simulink model "simulation"  (R2021b)
settings: Solver=ode15s  StartTime=0  StopTime=2474  RelTol=1e-4
model workspace: external: MATLAB File Z:\sleipner_simulation\data.m (data not in the file)
values from neighbouring files (symbols this model uses):
  AccessoryLoad = 200    [data.m]
  aeroDragCoeff = 0.38    [data.m]
  airDensity = 1.23    [data.m]
  C = 628.297    [data.m]
  driveLineGear = 3.55    [data.m]
  energyCapacity = 40    [data.m]
  frontArea = 16    [data.m]
  gravity = 9.82    [data.m]
  inertialMassVeh = 5000    [data.m]
  initialSOC = 0.95    [data.m]
  InternalResistance = 0.1    [data.m]
  kc = 0.0452    [data.m]
  ki = 0.0167    [data.m]
  kw = 5.664E-6    (= 5.664e-06)    [data.m]
  massVeh = 5000    [data.m]
  maxBreakForce = 10000    [data.m]
  motorModelMaxPowerOut = 10000    [data.m]
  motorModelMaxTrqOut = 600    [data.m]
  openCircuitVoltage = 396    [data.m]
  regenbreakFraction = 0.55    [data.m]
  rollingResistCoeff = 0.01    [data.m]
  spinLoss = 6    [data.m]
  wheelRadius = 0.35    [data.m]
undefined symbols (not defined in the file or in its folder): magnitude
libraries: simulink x5, slpidlib x1, autolibshared x1
settings Model: Creator=alexa  LastModifiedBy=alebostr
settings DebuggingCC: UnconnectedInputMsg=none  UnconnectedOutputMsg=none  UnconnectedLineMsg=none  UnderSpecifiedDimensionMsg=warning
settings ModelReferenceCC: EnableRefExpFcnMdlSchedulingChecks=off
settings RTWCC: DLArmComputeVersion=20.02.1

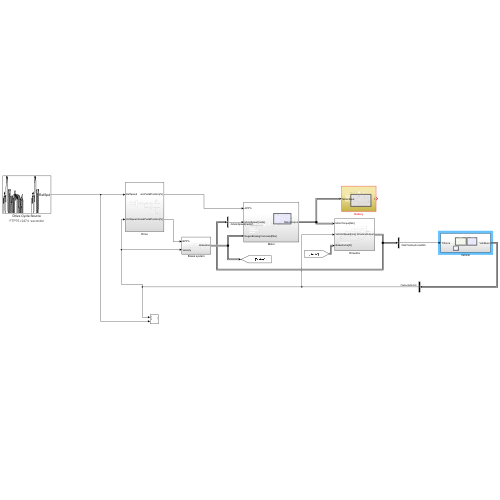
[thumbnail: Simulink's stored preview of the top-level diagram]
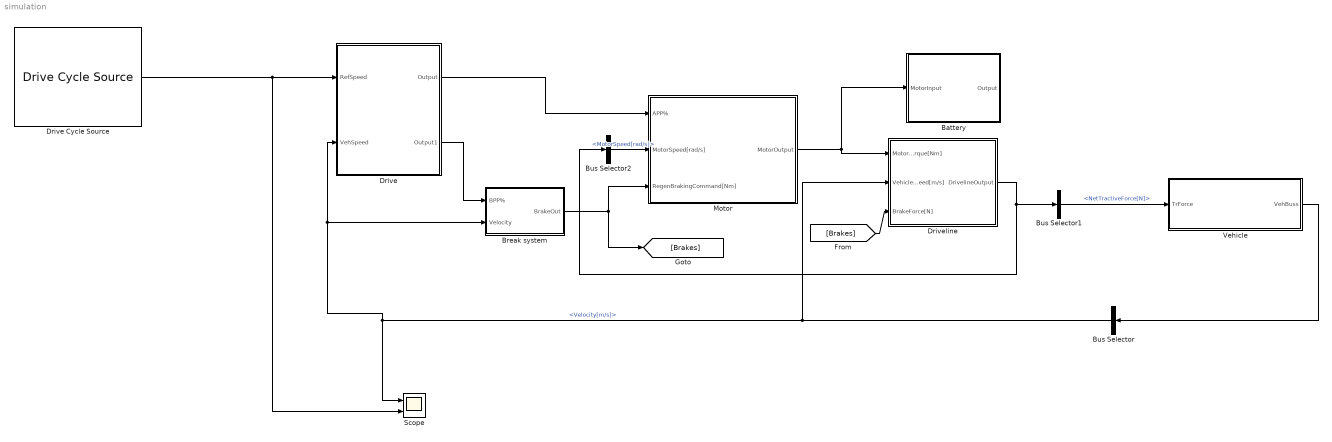
== system simulation ==
  Battery : Subsystem
  Break system : Subsystem
  Bus Selector : BusSelector  OutputSignals=Velocity[m/s]
  Bus Selector1 : BusSelector  OutputSignals=NetTractiveForce[N]
  Bus Selector2 : BusSelector  OutputSignals=MotorSpeed[rad/s]
  Drive : Subsystem
  Drive Cycle Source : autolibshared/Drive Cycle Source  cycleVar=FTP75  fileVar=cycleFTP75.mat  tfinal="2474  seconds"  cycleRepeat=off  outAccPort=off  outGearPort=off  gearList=No gear data  t_wot1=5  xdot_woto=0  xdot_wot1=30  t_wot2=20  xdot_wot2=0  t_wotend=30  srcUnit=m/s  outUnit=m/s  srcAccUnit=m/s/s  outAccUnit=m/s^2  dt=0  aMode=1  faultOption=off  velBnd=2  velBndUnit=mph  inUnit=m/s  timeBnd=1  failOption=off  stopSim=off  maxFaultCnt=10  maxFaultTime=2  maxTotFaultTime=15  traceOption=off  dtTrace=1  traceWindow=10  lastDCname=FTP75  lastOutUnit=mph  lastDT=0  lastTB=1  lastSB=2  forceCalcBound=off
      settings: SourceProductBaseCode=PW,DR,MT,UV,VE
  Driveline : Subsystem
  Motor : Subsystem
  Scope : Scope  NumInputPorts=2
  Vehicle : Subsystem
  wires:
  Drive/2(Output1) -> Break system/1(BPP%)
  Break system/1(BrakeOut) -> [Brakes], Motor/3(RegenBrakingCommand[Nm])
  Drive/1(Output) -> Motor/1(APP%)
  [Brakes] -> Driveline/3(BrakeForce[N])
  Motor/1(MotorOutput) -> Driveline/1(MotorTorque[Nm]), Battery/1(MotorInput)
  Driveline/1(DrivelineOutput) -> Bus Selector1/1, Bus Selector2/1
  Bus Selector2/1 -> Motor/2(MotorSpeed[rad/s])  "<MotorSpeed[rad/s]>"
  Vehicle/1(VehBuss) -> Bus Selector/1
  Bus Selector/1 -> Driveline/2(VehicleSpeed[m/s]), Drive/2(VehSpeed), Break system/2(Velocity), Scope/1  "<Velocity[m/s]>"
  Bus Selector1/1 -> Vehicle/1(TrForce)  "<NetTractiveForce[N]>"
  Drive Cycle Source/1 -> Scope/2, Drive/1(RefSpeed)

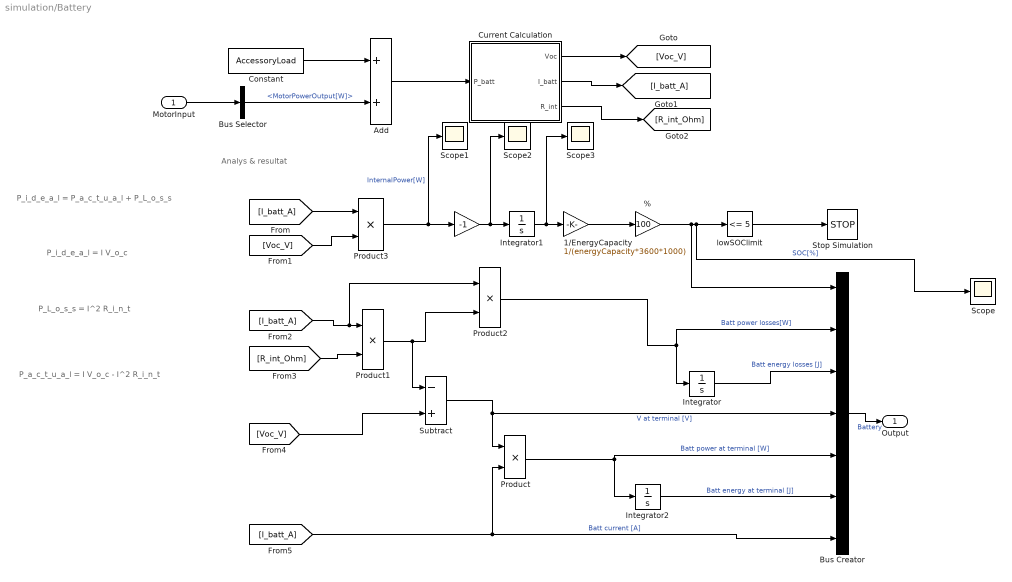
== system simulation/Battery ==
  note: Analys & resultat
  note: P_i_d_e_a_l = P_a_c_t_u_a_l + P_L_o_s_s
  note: P_a_c_t_u_a_l = I V_o_c - I^2 R_i_n_t
  note: P_i_d_e_a_l = I V_o_c
  note: P_L_o_s_s = I^2 R_i_n_t
  MotorInput : Inport
  " " : Gain  Gain=-1
  % : Gain  Gain=100
  1/EnergyCapacity : Gain  Gain=1/(energyCapacity*3600*1000)
  Add : Sum
  Bus Creator : BusCreator  Inputs=7
  Bus Selector : BusSelector  OutputSignals=MotorPowerOutput[W]
  Constant : Constant  Value=AccessoryLoad
  Current Calculation : Subsystem
  Integrator : Integrator
  Integrator1 : Integrator  InitialCondition=energyCapacity*3600*1000*initialSOC  IgnoreLimit=on
  Integrator2 : Integrator
  Product : Product
  Product1 : Product  RndMeth=Zero
  Product2 : Product  RndMeth=Zero
  Product3 : Product  RndMeth=Zero
  Scope{,1..3} (4 alike) : Scope
  Stop Simulation : Stop
  Subtract : Sum  Inputs=-+
  lowSOClimit : simulink/Logic and Bit Operations/Compare To Constant  relop=<=  const=5  OutDataTypeStr=boolean
  Output : Outport
  wires:
  MotorInput/1 -> Bus Selector/1
  Add/1 -> Current Calculation/1(P_batt)
  Constant/1 -> Add/1
  Current Calculation/1(" Voc") -> [Voc_V]
  Current Calculation/3(R_int) -> [R_int_Ohm]
  Current Calculation/2(I_batt) -> [I_batt_A]
  [I_batt_A] -> Product3/1
  [Voc_V] -> Product3/2
  Product3/1 -> Scope1/1, " "/1  "InternalPower[W]"
  " "/1 -> Scope2/1, Integrator1/1
  Integrator1/1 -> Scope3/1, 1/EnergyCapacity/1
  1/EnergyCapacity/1 -> %/1
  lowSOClimit/1 -> Stop Simulation/1
  %/1 -> Bus Creator/1, Scope/1, lowSOClimit/1  "SOC[%]"
  [I_batt_A] -> Product2/1, Product1/1
  [R_int_Ohm] -> Product1/2
  Product1/1 -> Subtract/1, Product2/2
  Product2/1 -> Integrator/1, Bus Creator/2  "Batt power losses[W]"
  Integrator/1 -> Bus Creator/3  "Batt energy losses [J]"
  [Voc_V] -> Subtract/2
  Subtract/1 -> Product/1, Bus Creator/4  "V at terminal [V]"
  [I_batt_A] -> Product/2, Bus Creator/7  "Batt current [A]"
  Product/1 -> Integrator2/1, Bus Creator/5  "Batt power at terminal [W]"
  Integrator2/1 -> Bus Creator/6  "Batt energy at terminal [J]"
  Bus Creator/1 -> Output/1  "Battery"
  Bus Selector/1 -> Add/2  "<MotorPowerOutput[W]>"

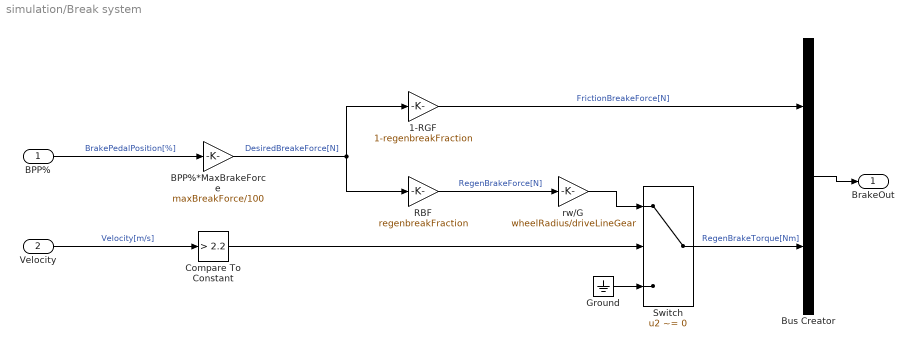
== system simulation/Break system ==
  BPP% : Inport
  Velocity : Inport  Port=2
  1-RGF : Gain  Gain=1-regenbreakFraction
  BPP%*MaxBrakeForce : Gain  Gain=maxBreakForce/100
  Bus Creator : BusCreator  Inputs=2
  Compare To Constant : simulink/Logic and Bit Operations/Compare To Constant  relop=>  const=2.2  OutDataTypeStr=boolean
  Ground : Ground
  RBF : Gain  Gain=regenbreakFraction
  Switch : Switch  Criteria=u2 ~= 0
  rw/G : Gain  Gain=wheelRadius/driveLineGear
  BrakeOut : Outport
  wires:
  1-RGF/1 -> Bus Creator/1  "FrictionBreakeForce[N]"
  rw/G/1 -> Switch/1
  Velocity/1 -> Compare To Constant/1  "Velocity[m/s]"
  Switch/1 -> Bus Creator/2  "RegenBrakeTorque[Nm]"
  BPP%*MaxBrakeForce/1 -> 1-RGF/1, RBF/1  "DesiredBreakeForce[N]"
  Bus Creator/1 -> BrakeOut/1
  RBF/1 -> rw/G/1  "RegenBrakeForce[N]"
  Compare To Constant/1 -> Switch/2
  BPP%/1 -> BPP%*MaxBrakeForce/1  "BrakePedalPosition[%]"
  Ground/1 -> Switch/3

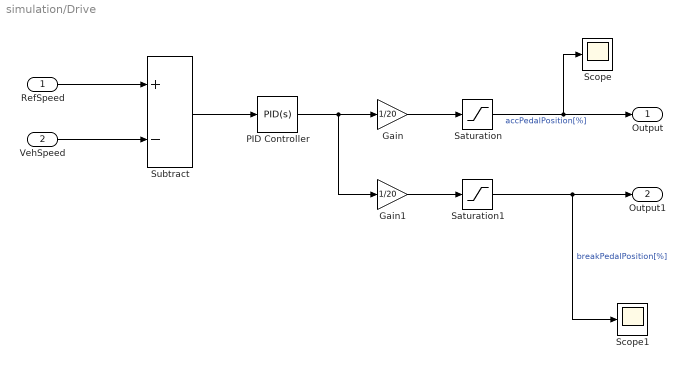
== system simulation/Drive ==
  RefSpeed : Inport
  VehSpeed : Inport  Port=2
  Gain : Gain  Gain=1/20
  Gain1 : Gain  Gain=1/20
  PID Controller : slpidlib/PID Controller  Controller=PID  Form=Parallel  TimeDomain=Continuous-time  UseExternalTs=off  SampleTime=-1  IntegratorMethod=Forward Euler  FilterMethod=Forward Euler  ControllerParametersSource=internal  P=200  I=1  D=0  UseFilter=on  N=100  TunerSelectOption=Transfer Function Based (PID Tuner App)  InitialConditionSource=internal  InitialConditionForIntegrator=0  InitialConditionForFilter=0  DifferentiatorICPrevScaledInput=0  ExternalReset=none  TrackingMode=off  Kt=1  LimitOutput=off  SatLimitsSource=internal  UpperSaturationLimit=inf  LowerSaturationLimit=-inf  LinearizeAsGain=on  AntiWindupMode=none  Kb=1  POutMin=[]  POutMax=[]  IOutMin=[]  IOutMax=[]  DOutMin=[]  DOutMax=[]  NOutMin=[]  NOutMax=[]  SumOutMin=[]  SumOutMax=[]  SaturationOutMin=[]  SaturationOutMax=[]  PParamMin=[]  PParamMax=[]  IParamMin=[]  IParamMax=[]  DParamMin=[]  DParamMax=[]  NParamMin=[]  NParamMax=[]  KbParamMin=[]  KbParamMax=[]  KtParamMin=[]  KtParamMax=[]  KbOutMin=[]  KbOutMax=[]  KtOutMin=[]  KtOutMax=[]  IntegratorOutMin=[]  IntegratorOutMax=[]  FilterOutMin=[]  FilterOutMax=[]  SumI1OutMin=[]  SumI1OutMax=[]  SumI2OutMin=[]  SumI2OutMax=[]  SumI3OutMin=[]  SumI3OutMax=[]  SumI4OutMin=[]  SumI4OutMax=[]  SumDOutMin=[]  SumDOutMax=[]  DifferentiatorOutMin=[]  DifferentiatorOutMax=[]  FilterDiffOutCoefMin=[]  FilterDiffOutCoefMax=[]  ReciprocalOutMin=[]  ReciprocalOutMax=[]  SumDenOutMin=[]  SumDenOutMax=[]  SumNumOutMin=[]  SumNumOutMax=[]  DivideOutMin=[]  DivideOutMax=[]  UdiffTsProdOutMin=[]  UdiffTsProdOutMax=[]  NTsProdOutMin=[]  NTsProdOutMax=[]  UintegralTsProdOutMin=[]  UintegralTsProdOutMax=[]  UngainTsProdOutMin=[]  UngainTsProdOutMax=[]  IntegratorContinuousStateAttributes=''  IntegratorStateMustResolveToSignalObject=off  IntegratorRTWStateStorageClass=Auto  FilterContinuousStateAttributes=''  FilterStateMustResolveToSignalObject=off  FilterRTWStateStorageClass=Auto  ParallelPVariant=InternalParameters  IdealPVariant=Disabled  IVariant=InternalParameters  DVariant=InternalParameters  IntegratorVariant=Continuous  SatVariant=Disabled  AWVariant=Passthrough  PCopyVariant=Disabled  TRVariant=Disabled  FdbkBlocksVariant=Forward  IdealPFdbkVariant=Disabled  SatFdbkVariant=Disabled  DerivativeFilterVariant=ContFilter  NVariant=InternalParameters  NCopyVariant=Disabled  FilterICVariant=InternalICsFilter  IntegratorICVariant=InternalICs  ExternalResetVariant=Disabled  TRSumVariant=Passthrough  SumFdbkVariant=Disabled  SumVariant=Sum_PID  TsampFilterVariant=InternalTs  TsampNgainVariant=Passthrough  TsampIntegralVariant=Passthrough  ExternalSaturationOutDataTypeStr=Inherit: Same as second input
  Saturation : Saturate  UpperLimit=100  LowerLimit=0  ZeroCross=off
  Saturation1 : Saturate  UpperLimit=0  LowerLimit=-100  ZeroCross=off
  Scope : Scope
  Scope1 : Scope
  Subtract : Sum  Inputs=+-
  Output : Outport
  Output1 : Outport  Port=2
  wires:
  RefSpeed/1 -> Subtract/1
  VehSpeed/1 -> Subtract/2
  Saturation/1 -> Scope/1, Output/1  "accPedalPosition[%]"
  Saturation1/1 -> Scope1/1, Output1/1  "breakPedalPosition[%]"
  Gain/1 -> Saturation/1
  Gain1/1 -> Saturation1/1
  Subtract/1 -> PID Controller/1
  PID Controller/1 -> Gain1/1, Gain/1

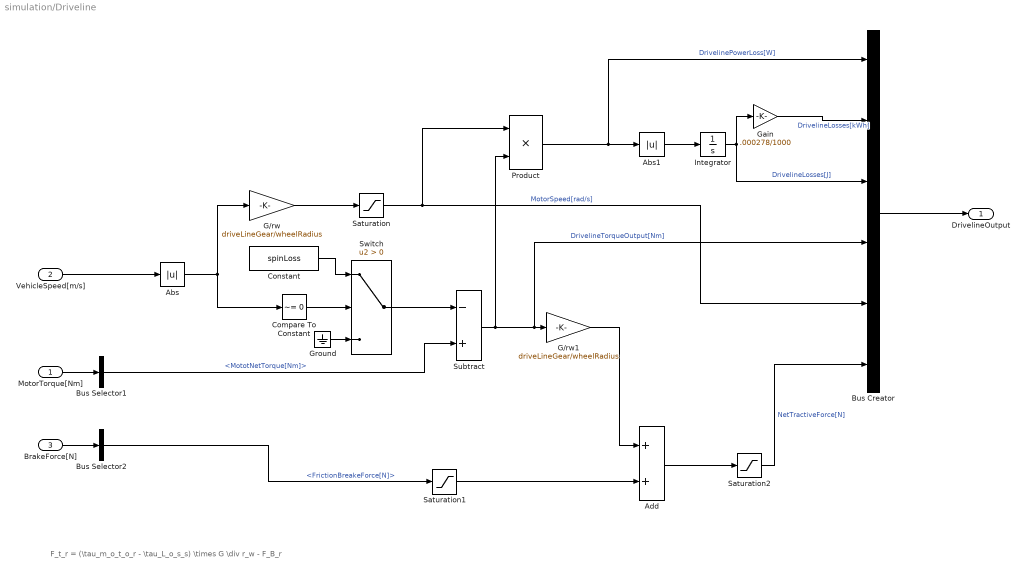
== system simulation/Driveline ==
  note: F_t_r = (\tau_m_o_t_o_r - \tau_L_o_s_s) \times G \div r_w - F_B_r
  MotorTorque[Nm] : Inport
  VehicleSpeed[m/s] : Inport  Port=2
  BrakeForce[N] : Inport  Port=3
  Abs : Abs
  Abs1 : Abs
  Add : Sum
  Bus Creator : BusCreator  Inputs=6
  Bus Selector1 : BusSelector  OutputSignals=MototNetTorque[Nm]
  Bus Selector2 : BusSelector  OutputSignals=FrictionBreakeForce[N]
  Compare To Constant : simulink/Logic and Bit Operations/Compare To Constant  relop=~=  const=0  OutDataTypeStr=boolean
  Constant : Constant  Value=spinLoss
  G/rw : Gain  Gain=driveLineGear/wheelRadius
  G/rw1 : Gain  Gain=driveLineGear/wheelRadius
  Gain : Gain  Gain=.000278/1000
  Ground : Ground
  Integrator : Integrator
  Product : Product
  Saturation : Saturate  UpperLimit=inf  LowerLimit=0.00001
  Saturation1 : Saturate  UpperLimit=0  LowerLimit=-10000
  Saturation2 : Saturate  UpperLimit=5000  LowerLimit=-10000
  Subtract : Sum  Inputs=-+
  Switch : Switch  Criteria=u2 > Threshold
  DrivelineOutput : Outport
  wires:
  Abs/1 -> G/rw/1, Compare To Constant/1
  G/rw/1 -> Saturation/1
  Constant/1 -> Switch/1
  Ground/1 -> Switch/3
  Saturation/1 -> Bus Creator/5, Product/1  "MotorSpeed[rad/s]"
  Switch/1 -> Subtract/1
  Subtract/1 -> Bus Creator/4, G/rw1/1, Product/2  "DrivelineTorqueOutput[Nm]"
  G/rw1/1 -> Add/1
  Saturation1/1 -> Add/2
  Add/1 -> Saturation2/1
  Saturation2/1 -> Bus Creator/6  "NetTractiveForce[N]"
  Product/1 -> Abs1/1, Bus Creator/1  "DrivelinePowerLoss[W]"
  Abs1/1 -> Integrator/1
  Integrator/1 -> Gain/1, Bus Creator/3  "DrivelineLosses[J]"
  Gain/1 -> Bus Creator/2  "DrivelineLosses[kWh]"
  Bus Creator/1 -> DrivelineOutput/1
  VehicleSpeed[m/s]/1 -> Abs/1
  MotorTorque[Nm]/1 -> Bus Selector1/1
  Bus Selector1/1 -> Subtract/2  "<MototNetTorque[Nm]>"
  BrakeForce[N]/1 -> Bus Selector2/1
  Bus Selector2/1 -> Saturation1/1  "<FrictionBreakeForce[N]>"
  Compare To Constant/1 -> Switch/2

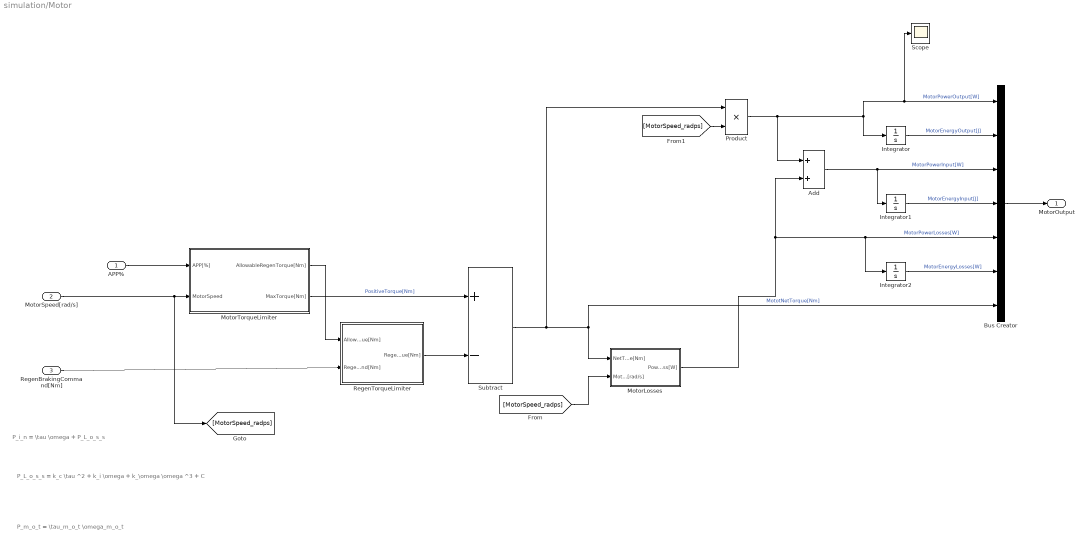
== system simulation/Motor ==
  note: P_i_n = \tau \omega + P_L_o_s_s
  note: P_m_o_t = \tau_m_o_t \omega_m_o_t
  note: P_L_o_s_s = k_c \tau ^2 + k_i \omega + k_\omega \omega ^3 + C
  APP% : Inport
  MotorSpeed[rad/s] : Inport  Port=2
  RegenBrakingCommand[Nm] : Inport  Port=3
  Add : Sum
  Bus Creator : BusCreator  Inputs=7
  Integrator : Integrator
  Integrator1 : Integrator
  Integrator2 : Integrator
  MotorLosses : Subsystem
  MotorTorqueLimiter : Subsystem
  Product : Product
  RegenTorqueLimiter : Subsystem
  Scope : Scope
  Subtract : Sum  Inputs=+-
  MotorOutput : Outport
  wires:
  APP%/1 -> MotorTorqueLimiter/1(APP[%])
  RegenBrakingCommand[Nm]/1 -> RegenTorqueLimiter/2(RegenBrakingCommand[Nm])
  MotorTorqueLimiter/1(AllowableRegenTorque[Nm]) -> RegenTorqueLimiter/1(AllowableRegenTorque[Nm])
  MotorTorqueLimiter/2(MaxTorque[Nm]) -> Subtract/1  "PositiveTorque[Nm]"
  RegenTorqueLimiter/1(RegenTorque[Nm]) -> Subtract/2
  Subtract/1 -> Product/1, MotorLosses/1(NetTorque[Nm]), Bus Creator/7  "MototNetTorque[Nm]"
  [MotorSpeed_radps] -> MotorLosses/2(MotorSpeed[rad/s])
  [MotorSpeed_radps] -> Product/2
  Product/1 -> Add/1, Scope/1, Bus Creator/1, Integrator/1  "MotorPowerOutput[W]"
  Integrator/1 -> Bus Creator/2  "MotorEnergyOutput[J]"
  MotorLosses/1(PowerLoss[W]) -> Integrator2/1, Bus Creator/5, Add/2  "MotorPowerLosses[W]"
  Add/1 -> Integrator1/1, Bus Creator/3  "MotorPowerInput[W]"
  Integrator1/1 -> Bus Creator/4  "MotorEnergyInput[J]"
  Integrator2/1 -> Bus Creator/6  "MotorEnergyLosses[W]"
  Bus Creator/1 -> MotorOutput/1
  MotorSpeed[rad/s]/1 -> [MotorSpeed_radps], MotorTorqueLimiter/2(MotorSpeed)

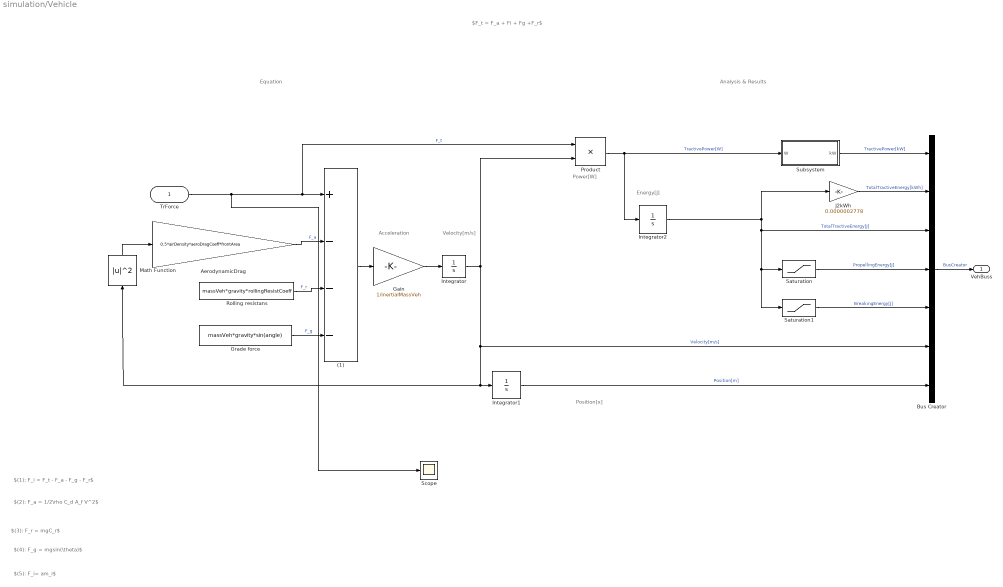
== system simulation/Vehicle ==
  note: $(1): F_i = F_t - F_a - F_g - F_r$
  note: Analysis & Results
  note: Power[W]
  note: Equation
  note: Velocity[m/s]
  note: Energy[J]
  note: Position[x]
  note: $F_t = F_a + Fi + Fg +F_r$
  note: Acceleration
  note: $(2): F_a = 1/2\rho C_d A_f V^2$
  note: $(3): F_r = mgC_r$
  note: $(4): F_g = mgsin(\theta)$
  note: $(5): F_i= am_i$
  TrForce : Inport
  (1) : Sum  Inputs=+---
  AerodynamicDrag : Gain  Gain=0.5*airDensity*aeroDragCoeff*frontArea
  Bus Creator : BusCreator  Inputs=7
  Gain : Gain  Gain=1/inertialMassVeh
  Grade force : Constant  Value=massVeh*gravity*sin(angle)
  Integrator : Integrator  LowerSaturationLimit=0.0001
  Integrator1 : Integrator
  Integrator2 : Integrator
  J2kWh : Gain  Gain=0.0000002778
  Math Function : Math  Operator=magnitude^2  SaturateOnIntegerOverflow=on
  Product : Product
  Rolling resistans : Constant  Value=massVeh*gravity*rollingResistCoeff
  Saturation : Saturate  UpperLimit=inf  LowerLimit=0
  Saturation1 : Saturate  UpperLimit=0  LowerLimit=-inf
  Scope : Scope
  Subsystem : Subsystem
  VehBuss : Outport
  wires:
  (1)/1 -> Gain/1
  AerodynamicDrag/1 -> (1)/2  "F_a"
  Gain/1 -> Integrator/1
  Math Function/1 -> AerodynamicDrag/1
  TrForce/1 -> Scope/1, Product/1, (1)/1  "F_t"
  Saturation/1 -> Bus Creator/4  "PropellingEnergy[J]"
  Integrator1/1 -> Bus Creator/7  "Position[m]"
  Grade force/1 -> (1)/4  "F_g"
  Saturation1/1 -> Bus Creator/5  "BreakingEnergy[J]"
  Rolling resistans/1 -> (1)/3  "F_r"
  Integrator2/1 -> J2kWh/1, Saturation1/1, Saturation/1, Bus Creator/3  "TotalTractiveEnergy[J]"
  J2kWh/1 -> Bus Creator/2  "TotalTractiveEnergy[kWh]"
  Bus Creator/1 -> VehBuss/1  "BusCreator"
  Product/1 -> Subsystem/1(W), Integrator2/1  "TractivePower[W]"
  Subsystem/1(kW) -> Bus Creator/1  "TractivePower[kW]"
  Integrator/1 -> Bus Creator/6, Integrator1/1, Math Function/1, Product/2  "Velocity[m/s]"

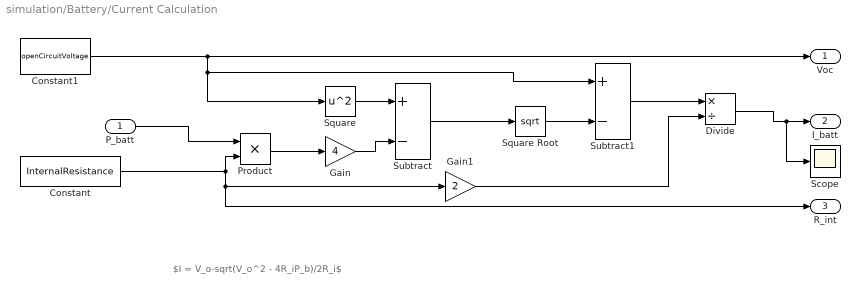
== system simulation/Battery/Current Calculation ==
  note: $I = V_o-sqrt(V_o^2 - 4R_iP_b)/2R_i$
  P_batt : Inport
  Constant : Constant  Value=InternalResistance
  Constant1 : Constant  Value=openCircuitVoltage
  Divide : Product  Inputs=*/
  Gain : Gain  Gain=4
  Gain1 : Gain  Gain=2
  Product : Product
  Scope : Scope
  Square : Math  Operator=square  SaturateOnIntegerOverflow=on
  Square Root : Sqrt  SaturateOnIntegerOverflow=on
  Subtract : Sum  Inputs=+-
  Subtract1 : Sum  Inputs=+-
  " Voc" : Outport
  I_batt : Outport  Port=2
  R_int : Outport  Port=3
  wires:
  P_batt/1 -> Product/1
  Constant/1 -> Product/2, Gain1/1, R_int/1
  Product/1 -> Gain/1
  Constant1/1 -> Square/1, Subtract1/1, " Voc"/1
  Square/1 -> Subtract/1
  Gain/1 -> Subtract/2
  Subtract/1 -> Square Root/1
  Square Root/1 -> Subtract1/2
  Subtract1/1 -> Divide/1
  Gain1/1 -> Divide/2
  Divide/1 -> Scope/1, I_batt/1

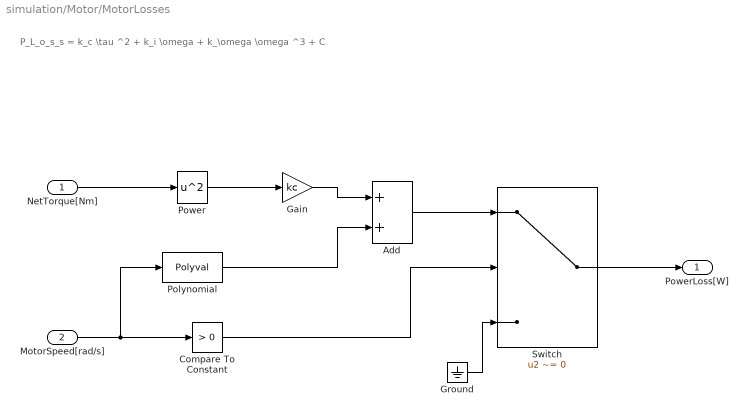
== system simulation/Motor/MotorLosses ==
  note: P_L_o_s_s = k_c \tau ^2 + k_i \omega + k_\omega \omega ^3 + C
  NetTorque[Nm] : Inport
  MotorSpeed[rad/s] : Inport  Port=2
  Add : Sum
  Compare To Constant : simulink/Logic and Bit Operations/Compare To Constant  relop=>  const=0  OutDataTypeStr=boolean
  Gain : Gain  Gain=kc
  Ground : Ground
  Polynomial : Polyval  Coefs=[kw,0,ki,C]
  Power : Math  Operator=square  SaturateOnIntegerOverflow=on
  Switch : Switch  Criteria=u2 ~= 0
  PowerLoss[W] : Outport
  wires:
  NetTorque[Nm]/1 -> Power/1
  Power/1 -> Gain/1
  Gain/1 -> Add/1
  Polynomial/1 -> Add/2
  Add/1 -> Switch/1
  Compare To Constant/1 -> Switch/2
  Switch/1 -> PowerLoss[W]/1
  Ground/1 -> Switch/3
  MotorSpeed[rad/s]/1 -> Polynomial/1, Compare To Constant/1

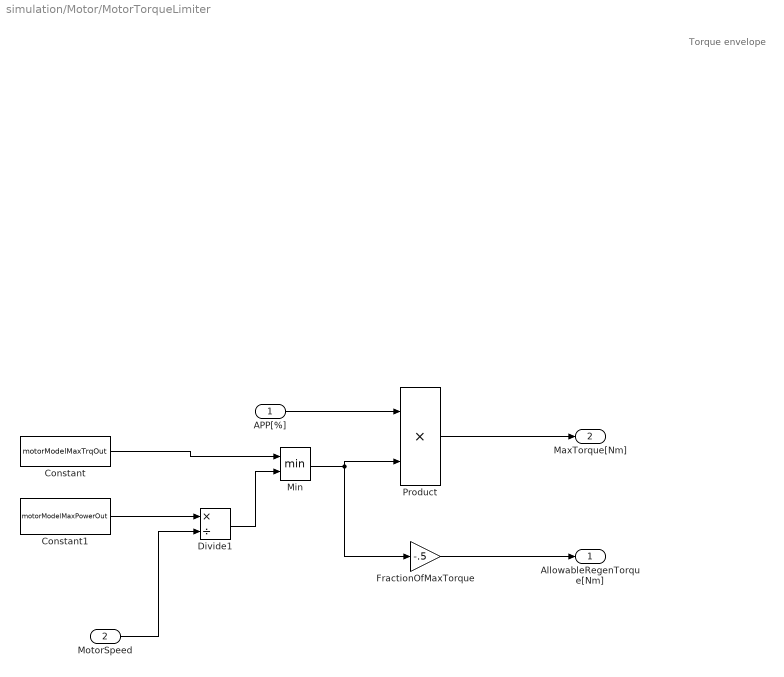
== system simulation/Motor/MotorTorqueLimiter ==
  note: Torque envelope
  APP[%] : Inport
  MotorSpeed : Inport  Port=2
  Constant : Constant  Value=motorModelMaxTrqOut
  Constant1 : Constant  Value=motorModelMaxPowerOut
  Divide1 : Product  Inputs=*/
  FractionOfMaxTorque : Gain  Gain=-.5
  Min : MinMax  Inputs=2
  Product : Product
  AllowableRegenTorque[Nm] : Outport
  MaxTorque[Nm] : Outport  Port=2
  wires:
  Constant1/1 -> Divide1/1
  MotorSpeed/1 -> Divide1/2
  Constant/1 -> Min/1
  Divide1/1 -> Min/2
  Min/1 -> Product/2, FractionOfMaxTorque/1
  APP[%]/1 -> Product/1
  FractionOfMaxTorque/1 -> AllowableRegenTorque[Nm]/1
  Product/1 -> MaxTorque[Nm]/1

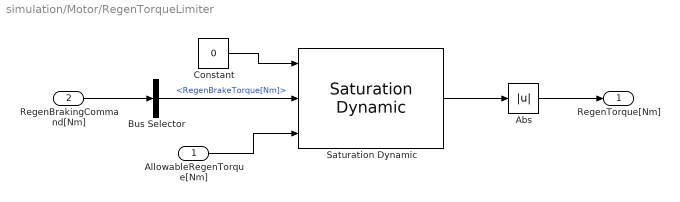
== system simulation/Motor/RegenTorqueLimiter ==
  AllowableRegenTorque[Nm] : Inport
  RegenBrakingCommand[Nm] : Inport  Port=2
  Abs : Abs
  Bus Selector : BusSelector  OutputSignals=RegenBrakeTorque[Nm]
  Constant : Constant  Value=0
  Saturation Dynamic : simulink/Discontinuities/Saturation Dynamic  OutMin=[]  OutMax=[]  OutDataTypeStr=Inherit: Same as second input  OutDataType=fixdt(1, 16)  OutScaling=2^-10  DoSatur=off
  RegenTorque[Nm] : Outport
  wires:
  RegenBrakingCommand[Nm]/1 -> Bus Selector/1
  Constant/1 -> Saturation Dynamic/1
  Bus Selector/1 -> Saturation Dynamic/2  "<RegenBrakeTorque[Nm]>"
  AllowableRegenTorque[Nm]/1 -> Saturation Dynamic/3
  Saturation Dynamic/1 -> Abs/1
  Abs/1 -> RegenTorque[Nm]/1

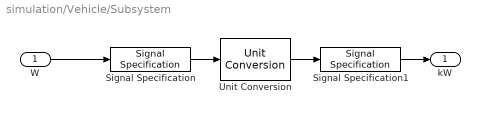
== system simulation/Vehicle/Subsystem ==
  W : Inport
  Signal Specification : SignalSpecification  Unit=W
  Signal Specification1 : SignalSpecification  Unit=kW
  Unit Conversion : UnitConversion
  kW : Outport
  wires:
  W/1 -> Signal Specification/1
  Signal Specification/1 -> Unit Conversion/1
  Unit Conversion/1 -> Signal Specification1/1
  Signal Specification1/1 -> kW/1
